simulink model "doa_no_gotos"  (R2013b)
settings: Solver=ode45  StartTime=0.0  StopTime=10.0  RelTol=1e-3
undefined symbols (not defined in the file or in its folder): calan_lib, comp_addsub
libraries: xbsIndex_r4 x1532, casper_library_misc x168, casper_library_delays x24
(part 1 of 16)
settings Model: Creator=root  LastModifiedBy=root

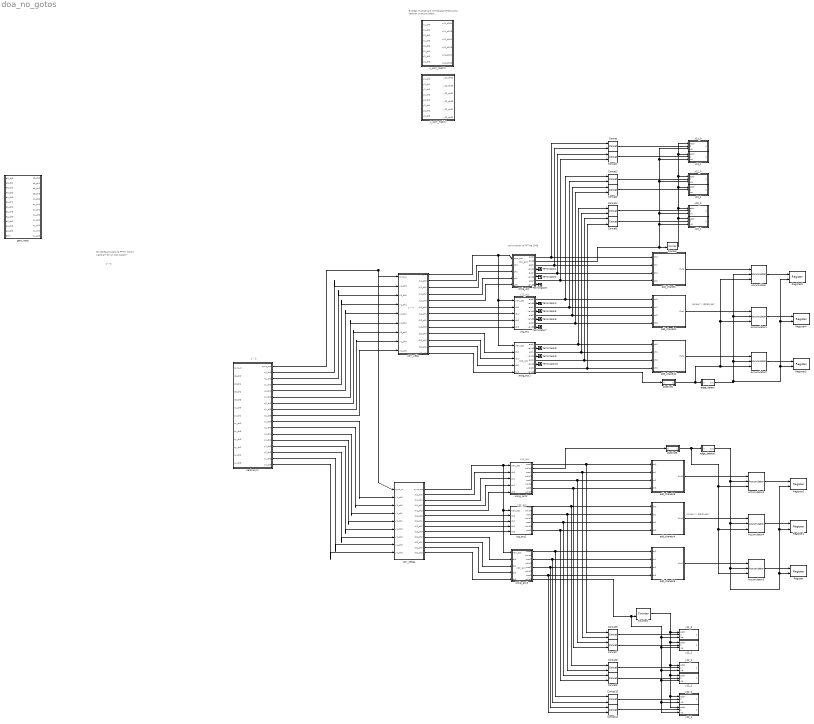
== system doa_no_gotos ==
  note: review!!! datatype!!
  note: x11_acc
  note: x12_acc
  note: x22_acc
  note: voy a tomar la FFT de 2048
  note: z^-7
  note: z^-2
  note: El diego multiplica e inmediatamente suma
      | todo en un acumulador..
  note: z^-3
  note: Es necesario para la FFT??
      | Como calibrar? en un solo canal??
  note: x11_acc
  note: x12_acc
  note: x22_acc
  note: review!!! datatype!!
  Accumulator{,1..5} (6 alike) : xbsIndex_r4/Accumulator  operation=Add  n_bits=64  overflow=Saturate  scale=1  rst=on  infoeditControl=reset for floating point data type must be asserted for a minimum of 2 cycles  hasbypass=off  en=on  latency=0  dbl_ovrd=off  msb_inp=100  msb=100  lsb=-100  use_behavioral_HDL=on  implementation=Fabric  block_type=accum
  Concat{,1..11} (12 alike) : xbsIndex_r4/Concat  num_inputs=2  dbl_ovrd=off  block_type=concat
  Counter : xbsIndex_r4/Counter  cnt_type=Free Running  cnt_to=Inf  operation=Up  start_count=0  cnt_by_val=1  arith_type=Unsigned  n_bits=9  bin_pt=0  load_pin=off  rst=on  en=on  explicit_period=on  period=1  dbl_ovrd=off  use_behavioral_HDL=off  implementation=Fabric  block_type=counter
  Counter1 : xbsIndex_r4/Counter  cnt_type=Free Running  cnt_to=Inf  operation=Up  start_count=0  cnt_by_val=1  arith_type=Unsigned  n_bits=9  bin_pt=0  load_pin=off  rst=on  en=on  explicit_period=on  period=1  dbl_ovrd=off  use_behavioral_HDL=off  implementation=Fabric  block_type=counter
  Register{,1..5} (6 alike) : xbsIndex_r4/Register  init=0  rst=off  en=on  dbl_ovrd=off  block_type=register
  Terminator{1..10} (10 alike) : Terminator
  add_chanels : Subsystem
  add_chanels1 : Subsystem
  add_chanels2 : Subsystem
  add_chanels3 : Subsystem
  add_chanels4 : Subsystem
  add_chanels5 : Subsystem
  centrosym : Subsystem
  corr_seba : Subsystem
  corr_seba1 : Subsystem
  edge_detect : Subsystem  AncestorBlock=casper_library_misc/edge_detect  mask(edge_detect){edge=Falling, polarity=Active High, x_in=[0 0.08 0.08 0.16 0.16 0.24 0.24 0.32 0.32 0.4], y_in=[-1 -1  1  1  1  1  1  1  1  1], x_out=[0.6 0.68 0.68 0.76 0.76 0.84 0.84 0.92 0.92 1], y_out=[-1 -1  1  1 -1 -1 -1 -1 -1 -1]}
      mask prompts: edge "Edge Type"; polarity "Output Polarity"; x_in "Input X Positions"; y_in "Input Y Positions"; x_out "Output X Positions"; y_out "Output Y Positions"
      mask help: Output is active for one-cycle after each edge of the specified type (i.e. rising, falling or both).
      mask init:
      | edge_detect_init(gcb,...
      |     'edge',edge,...
      |     'polarity',polarity,...
      |     'x_in',x_in,...
      |     'x_out',x_out,...
      |     'y_in',y_in,...
      |     'y_out',y_out);
      | 
      | x_in_num=str2num(getfield(getfield(get_param(gcb,'UserData'),'parameters'),'x_in'));
      | x_out_num=str2num(getfield(getfield(get_param(gcb,'UserData'),'parameters'),'x_out'));
      | y_in_num=str2num(getfield(getfield(get_param(gcb,'UserData'),'parameters'),'y_in'));
      | y_out_num=str2num(getfield(getfield(get_param(gcb,'UserData'),'parameters'),'y_out'));
      settings: AttributesFormatString=|
      | falling edges
      | active high
      mask Help: Output is active for one-cycle after each edge of the specified type (i.e. rising, falling, or both).  Latency is zero.
      mask TypeOptions edge: Rising | Falling | Both
      mask TypeOptions polarity: Active High | Active Low
      mask Display:
      | plot(x_in_num,0.5+y_in_num*0.2);
      | plot(x_out_num,0.5+y_out_num*0.2);
  edge_detect1 : Subsystem  AncestorBlock=casper_library_misc/edge_detect  mask(edge_detect){edge=Falling, polarity=Active High, x_in=[0 0.08 0.08 0.16 0.16 0.24 0.24 0.32 0.32 0.4], y_in=[-1 -1  1  1  1  1  1  1  1  1], x_out=[0.6 0.68 0.68 0.76 0.76 0.84 0.84 0.92 0.92 1], y_out=[-1 -1  1  1 -1 -1 -1 -1 -1 -1]}
      mask prompts: edge "Edge Type"; polarity "Output Polarity"; x_in "Input X Positions"; y_in "Input Y Positions"; x_out "Output X Positions"; y_out "Output Y Positions"
      mask help: Output is active for one-cycle after each edge of the specified type (i.e. rising, falling or both).
      mask init: same as doa_no_gotos/edge_detect
      settings: AttributesFormatString=|
      | falling edges
      | active high
      mask Help: Output is active for one-cycle after each edge of the specified type (i.e. rising, falling, or both).  Latency is zero.
      mask TypeOptions edge: Rising | Falling | Both
      mask TypeOptions polarity: Active High | Active Low
      mask Display:
      | plot(x_in_num,0.5+y_in_num*0.2);
      | plot(x_out_num,0.5+y_out_num*0.2);
  gain_input : Subsystem
  pipeline1 : Subsystem  AncestorBlock=casper_library_delays/pipeline  mask(pipeline){latency=9}
      mask help:
      | An explicitly laid-out delay line to avoid mapping to SRL16s
      | for use in pipelining to help achieve timing closure.
      mask init:
      | pipeline_init(gcb,'latency',latency);
      settings: AttributesFormatString=Latency = %<latency>
      mask Display:
      | port_label('input', 1, 'd');
      | port_label('output', 1, 'q');
      | disp(['Z^-', num2str(latency)]);
  pipeline5 : Subsystem  AncestorBlock=casper_library_delays/pipeline  mask(pipeline){latency=9}
      mask help:
      | An explicitly laid-out delay line to avoid mapping to SRL16s
      | for use in pipelining to help achieve timing closure.
      mask init:
      | pipeline_init(gcb,'latency',latency);
      settings: AttributesFormatString=Latency = %<latency>
      mask Display:
      | port_label('input', 1, 'd');
      | port_label('output', 1, 'q');
      | disp(['Z^-', num2str(latency)]);
  sig_acc : Subsystem
  sig_acc1 : Subsystem
  unsig_acc : Subsystem
  unsig_acc1 : Subsystem
  unsig_acc2 : Subsystem
  unsig_acc3 : Subsystem
  x11_0 : Subsystem  Tag=xps:bram  AncestorBlock=xps_library/Shared_BRAM  mask{arith_type=Unsigned, addr_width=9, data_width=64, reg_prim_output=off, reg_core_output=off, optimization=Minimum_Area, data_bin_pt=0, init_vals=[0:2^10-1], sample_rate=1}
      mask prompts: arith_type "Output Data Type"; addr_width "Address width"; data_width "Data Width"; reg_prim_output "Register Primitive Output"; reg_core_output "Register Core Output"; data_bin_pt "Data Binary Point"; init_vals "Initial values (simulation only)"; sample_rate "Sample rate"
      mask init:
      | shared_bram_mask;
      mask TypeOptions arith_type: Unsigned | Signed  (2's comp)
      mask TypeOptions data_width: 8 | 16 | 32 | 64 | 128
      mask TypeOptions optimization: Minimum_Area | Low_Power
  x11_1 : Subsystem  Tag=xps:bram  AncestorBlock=xps_library/Shared_BRAM  mask{arith_type=Unsigned, addr_width=9, data_width=64, reg_prim_output=off, reg_core_output=off, optimization=Minimum_Area, data_bin_pt=0, init_vals=[0:2^10-1], sample_rate=1}
      mask prompts: arith_type "Output Data Type"; addr_width "Address width"; data_width "Data Width"; reg_prim_output "Register Primitive Output"; reg_core_output "Register Core Output"; data_bin_pt "Data Binary Point"; init_vals "Initial values (simulation only)"; sample_rate "Sample rate"
      mask init:
      | shared_bram_mask;
      mask TypeOptions arith_type: Unsigned | Signed  (2's comp)
      mask TypeOptions data_width: 8 | 16 | 32 | 64 | 128
      mask TypeOptions optimization: Minimum_Area | Low_Power
  x12_0 : Subsystem  Tag=xps:bram  AncestorBlock=xps_library/Shared_BRAM  mask{arith_type=Unsigned, addr_width=9, data_width=64, reg_prim_output=off, reg_core_output=off, optimization=Minimum_Area, data_bin_pt=0, init_vals=[0:2^10-1], sample_rate=1}
      mask prompts: arith_type "Output Data Type"; addr_width "Address width"; data_width "Data Width"; reg_prim_output "Register Primitive Output"; reg_core_output "Register Core Output"; data_bin_pt "Data Binary Point"; init_vals "Initial values (simulation only)"; sample_rate "Sample rate"
      mask init:
      | shared_bram_mask;
      mask TypeOptions arith_type: Unsigned | Signed  (2's comp)
      mask TypeOptions data_width: 8 | 16 | 32 | 64 | 128
      mask TypeOptions optimization: Minimum_Area | Low_Power
  x12_1 : Subsystem  Tag=xps:bram  AncestorBlock=xps_library/Shared_BRAM  mask{arith_type=Unsigned, addr_width=9, data_width=64, reg_prim_output=off, reg_core_output=off, optimization=Minimum_Area, data_bin_pt=0, init_vals=[0:2^10-1], sample_rate=1}
      mask prompts: arith_type "Output Data Type"; addr_width "Address width"; data_width "Data Width"; reg_prim_output "Register Primitive Output"; reg_core_output "Register Core Output"; data_bin_pt "Data Binary Point"; init_vals "Initial values (simulation only)"; sample_rate "Sample rate"
      mask init:
      | shared_bram_mask;
      mask TypeOptions arith_type: Unsigned | Signed  (2's comp)
      mask TypeOptions data_width: 8 | 16 | 32 | 64 | 128
      mask TypeOptions optimization: Minimum_Area | Low_Power
  x22_0 : Subsystem  Tag=xps:bram  AncestorBlock=xps_library/Shared_BRAM  mask{arith_type=Unsigned, addr_width=9, data_width=64, reg_prim_output=off, reg_core_output=off, optimization=Minimum_Area, data_bin_pt=0, init_vals=[0:2^10-1], sample_rate=1}
      mask prompts: arith_type "Output Data Type"; addr_width "Address width"; data_width "Data Width"; reg_prim_output "Register Primitive Output"; reg_core_output "Register Core Output"; data_bin_pt "Data Binary Point"; init_vals "Initial values (simulation only)"; sample_rate "Sample rate"
      mask init:
      | shared_bram_mask;
      mask TypeOptions arith_type: Unsigned | Signed  (2's comp)
      mask TypeOptions data_width: 8 | 16 | 32 | 64 | 128
      mask TypeOptions optimization: Minimum_Area | Low_Power
  x22_1 : Subsystem  Tag=xps:bram  AncestorBlock=xps_library/Shared_BRAM  mask{arith_type=Unsigned, addr_width=9, data_width=64, reg_prim_output=off, reg_core_output=off, optimization=Minimum_Area, data_bin_pt=0, init_vals=[0:2^10-1], sample_rate=1}
      mask prompts: arith_type "Output Data Type"; addr_width "Address width"; data_width "Data Width"; reg_prim_output "Register Primitive Output"; reg_core_output "Register Core Output"; data_bin_pt "Data Binary Point"; init_vals "Initial values (simulation only)"; sample_rate "Sample rate"
      mask init:
      | shared_bram_mask;
      mask TypeOptions arith_type: Unsigned | Signed  (2's comp)
      mask TypeOptions data_width: 8 | 16 | 32 | 64 | 128
      mask TypeOptions optimization: Minimum_Area | Low_Power
  x_corr_matrix : Subsystem
  y11_0 : Subsystem  Tag=xps:bram  AncestorBlock=xps_library/Shared_BRAM  mask{arith_type=Unsigned, addr_width=9, data_width=64, reg_prim_output=off, reg_core_output=off, optimization=Minimum_Area, data_bin_pt=0, init_vals=[0:2^10-1], sample_rate=1}
      mask prompts: arith_type "Output Data Type"; addr_width "Address width"; data_width "Data Width"; reg_prim_output "Register Primitive Output"; reg_core_output "Register Core Output"; data_bin_pt "Data Binary Point"; init_vals "Initial values (simulation only)"; sample_rate "Sample rate"
      mask init:
      | shared_bram_mask;
      mask TypeOptions arith_type: Unsigned | Signed  (2's comp)
      mask TypeOptions data_width: 8 | 16 | 32 | 64 | 128
      mask TypeOptions optimization: Minimum_Area | Low_Power
  y11_1 : Subsystem  Tag=xps:bram  AncestorBlock=xps_library/Shared_BRAM  mask{arith_type=Unsigned, addr_width=9, data_width=64, reg_prim_output=off, reg_core_output=off, optimization=Minimum_Area, data_bin_pt=0, init_vals=[0:2^10-1], sample_rate=1}
      mask prompts: arith_type "Output Data Type"; addr_width "Address width"; data_width "Data Width"; reg_prim_output "Register Primitive Output"; reg_core_output "Register Core Output"; data_bin_pt "Data Binary Point"; init_vals "Initial values (simulation only)"; sample_rate "Sample rate"
      mask init:
      | shared_bram_mask;
      mask TypeOptions arith_type: Unsigned | Signed  (2's comp)
      mask TypeOptions data_width: 8 | 16 | 32 | 64 | 128
      mask TypeOptions optimization: Minimum_Area | Low_Power
  y12_0 : Subsystem  Tag=xps:bram  AncestorBlock=xps_library/Shared_BRAM  mask{arith_type=Unsigned, addr_width=9, data_width=64, reg_prim_output=off, reg_core_output=off, optimization=Minimum_Area, data_bin_pt=0, init_vals=[0:2^10-1], sample_rate=1}
      mask prompts: arith_type "Output Data Type"; addr_width "Address width"; data_width "Data Width"; reg_prim_output "Register Primitive Output"; reg_core_output "Register Core Output"; data_bin_pt "Data Binary Point"; init_vals "Initial values (simulation only)"; sample_rate "Sample rate"
      mask init:
      | shared_bram_mask;
      mask TypeOptions arith_type: Unsigned | Signed  (2's comp)
      mask TypeOptions data_width: 8 | 16 | 32 | 64 | 128
      mask TypeOptions optimization: Minimum_Area | Low_Power
  y12_1 : Subsystem  Tag=xps:bram  AncestorBlock=xps_library/Shared_BRAM  mask{arith_type=Unsigned, addr_width=9, data_width=64, reg_prim_output=off, reg_core_output=off, optimization=Minimum_Area, data_bin_pt=0, init_vals=[0:2^10-1], sample_rate=1}
      mask prompts: arith_type "Output Data Type"; addr_width "Address width"; data_width "Data Width"; reg_prim_output "Register Primitive Output"; reg_core_output "Register Core Output"; data_bin_pt "Data Binary Point"; init_vals "Initial values (simulation only)"; sample_rate "Sample rate"
      mask init:
      | shared_bram_mask;
      mask TypeOptions arith_type: Unsigned | Signed  (2's comp)
      mask TypeOptions data_width: 8 | 16 | 32 | 64 | 128
      mask TypeOptions optimization: Minimum_Area | Low_Power
  y22_0 : Subsystem  Tag=xps:bram  AncestorBlock=xps_library/Shared_BRAM  mask{arith_type=Unsigned, addr_width=9, data_width=64, reg_prim_output=off, reg_core_output=off, optimization=Minimum_Area, data_bin_pt=0, init_vals=[0:2^10-1], sample_rate=1}
      mask prompts: arith_type "Output Data Type"; addr_width "Address width"; data_width "Data Width"; reg_prim_output "Register Primitive Output"; reg_core_output "Register Core Output"; data_bin_pt "Data Binary Point"; init_vals "Initial values (simulation only)"; sample_rate "Sample rate"
      mask init:
      | shared_bram_mask;
      mask TypeOptions arith_type: Unsigned | Signed  (2's comp)
      mask TypeOptions data_width: 8 | 16 | 32 | 64 | 128
      mask TypeOptions optimization: Minimum_Area | Low_Power
  y22_1 : Subsystem  Tag=xps:bram  AncestorBlock=xps_library/Shared_BRAM  mask{arith_type=Unsigned, addr_width=9, data_width=64, reg_prim_output=off, reg_core_output=off, optimization=Minimum_Area, data_bin_pt=0, init_vals=[0:2^10-1], sample_rate=1}
      mask prompts: arith_type "Output Data Type"; addr_width "Address width"; data_width "Data Width"; reg_prim_output "Register Primitive Output"; reg_core_output "Register Core Output"; data_bin_pt "Data Binary Point"; init_vals "Initial values (simulation only)"; sample_rate "Sample rate"
      mask init:
      | shared_bram_mask;
      mask TypeOptions arith_type: Unsigned | Signed  (2's comp)
      mask TypeOptions data_width: 8 | 16 | 32 | 64 | 128
      mask TypeOptions optimization: Minimum_Area | Low_Power
  y_corr_matrix : Subsystem
  wires:
  corr_seba/5(r11_ch3) -> unsig_acc/5(ch3)
  corr_seba/2(r11_ch0) -> unsig_acc/2(ch0)
  corr_seba/4(r11_ch2) -> unsig_acc/4(ch2)
  corr_seba/3(r11_ch1) -> unsig_acc/3(ch1)
  corr_seba/1(sync_out) -> unsig_acc/1(new_acc), unsig_acc1/1(new_acc), sig_acc/1(new_acc)
  corr_seba/6(r12_ch0) -> sig_acc/2(ch0)
  corr_seba/7(r12_ch1) -> sig_acc/3(ch1)
  corr_seba/8(r12_ch2) -> sig_acc/4(ch2)
  corr_seba/9(r12_ch3) -> sig_acc/5(ch3)
  corr_seba/10(r22_ch0) -> unsig_acc1/2(ch0)
  corr_seba/13(r22_ch3) -> unsig_acc1/5(ch3)
  corr_seba/12(r22_ch2) -> unsig_acc1/4(ch2)
  corr_seba/11(r22_ch1) -> unsig_acc1/3(ch1)
  centrosym/1(sync_out) -> corr_seba1/1(sync_in), corr_seba/1(sync_in)
  centrosym/2(x1_ch0) -> corr_seba/2(x1_ch0)
  centrosym/3(x2_ch0) -> corr_seba/3(x2_ch0)
  centrosym/4(x1_ch1) -> corr_seba/4(x1_ch1)
  centrosym/5(x2_ch1) -> corr_seba/5(x2_ch1)
  centrosym/6(x1_ch2) -> corr_seba/6(x1_ch2)
  centrosym/7(x2_ch2) -> corr_seba/7(x2_ch2)
  centrosym/8(x1_ch3) -> corr_seba/8(x1_ch3)
  centrosym/9(x2_ch3) -> corr_seba/9(x2_ch3)
  corr_seba1/5(r11_ch3) -> unsig_acc2/5(ch3)
  corr_seba1/2(r11_ch0) -> unsig_acc2/2(ch0)
  corr_seba1/4(r11_ch2) -> unsig_acc2/4(ch2)
  corr_seba1/3(r11_ch1) -> unsig_acc2/3(ch1)
  corr_seba1/1(sync_out) -> unsig_acc3/1(new_acc), sig_acc1/1(new_acc), unsig_acc2/1(new_acc)
  corr_seba1/6(r12_ch0) -> sig_acc1/2(ch0)
  corr_seba1/7(r12_ch1) -> sig_acc1/3(ch1)
  corr_seba1/8(r12_ch2) -> sig_acc1/4(ch2)
  corr_seba1/9(r12_ch3) -> sig_acc1/5(ch3)
  corr_seba1/10(r22_ch0) -> unsig_acc3/2(ch0)
  corr_seba1/13(r22_ch3) -> unsig_acc3/5(ch3)
  corr_seba1/12(r22_ch2) -> unsig_acc3/4(ch2)
  corr_seba1/11(r22_ch1) -> unsig_acc3/3(ch1)
  centrosym/10(y1_ch0) -> corr_seba1/2(y1_ch0)
  centrosym/11(y2_ch0) -> corr_seba1/3(y2_ch0)
  centrosym/12(y1_ch1) -> corr_seba1/4(y1_ch1)
  centrosym/13(y2_ch1) -> corr_seba1/5(y2_ch1)
  centrosym/14(y1_ch2) -> corr_seba1/6(y1_ch2)
  centrosym/15(y2_ch2) -> corr_seba1/7(y2_ch2)
  centrosym/16(y1_ch3) -> corr_seba1/8(y1_ch3)
  centrosym/17(y2_ch3) -> corr_seba1/9(y2_ch3)
  pipeline1/1(q) -> edge_detect/1(in), Accumulator2/3, Accumulator1/3, Accumulator/3
  edge_detect/1(out) -> Register5/2, Register4/2, Register3/2, Accumulator2/2, Accumulator1/2, Accumulator/2
  unsig_acc1/8(valid3) -> pipeline1/1(d)
  unsig_acc/1(acc0) -> Concat/1, add_chanels/1(ch0)
  unsig_acc/3(acc1) -> Concat/2, add_chanels/2(ch1)
  unsig_acc/5(acc2) -> Concat1/1, add_chanels/3(ch2)
  unsig_acc/7(acc3) -> Concat1/2, add_chanels/4(ch3)
  add_chanels/1(Out1) -> Accumulator/1
  sig_acc/1(acc0) -> Concat2/1, add_chanels1/1(ch0)
  sig_acc/3(acc1) -> Concat2/2, add_chanels1/2(ch1)
  sig_acc/5(acc2) -> Concat3/1, add_chanels1/3(ch2)
  sig_acc/7(acc3) -> Concat3/2, add_chanels1/4(ch3)
  unsig_acc1/1(acc0) -> Concat4/1, add_chanels2/1(ch0)
  unsig_acc1/3(acc1) -> Concat4/2, add_chanels2/2(ch1)
  unsig_acc1/5(acc2) -> Concat5/1, add_chanels2/3(ch2)
  unsig_acc1/7(acc3) -> add_chanels2/4(ch3), Concat5/2
  add_chanels1/1(Out1) -> Accumulator1/1
  add_chanels2/1(Out1) -> Accumulator2/1
  unsig_acc/2(valid0) -> x22_0/3(we), x11_1/3(we), x11_0/3(we), x12_0/3(we), x22_1/3(we), Counter/2
  unsig_acc/4(valid1) -> Terminator1/1
  unsig_acc/6(valid2) -> Terminator2/1
  unsig_acc/8(valid3) -> Terminator3/1
  sig_acc/2(valid0) -> Terminator4/1
  sig_acc/4(valid1) -> Terminator5/1
  sig_acc/6(valid2) -> Terminator6/1
  sig_acc/8(valid3) -> Terminator7/1
  unsig_acc1/2(valid0) -> Terminator8/1
  unsig_acc1/4(valid1) -> Terminator9/1
  unsig_acc1/6(valid2) -> Terminator10/1
  pipeline5/1(q) -> Accumulator5/3, Accumulator4/3, Accumulator3/3, edge_detect1/1(in)
  edge_detect1/1(out) -> Register/2, Register1/2, Register2/2, Accumulator5/2, Accumulator4/2, Accumulator3/2
  unsig_acc2/2(valid0) -> pipeline5/1(d)
  unsig_acc2/1(acc0) -> Concat6/1, add_chanels3/1(ch0)
  unsig_acc2/3(acc1) -> Concat6/2, add_chanels3/2(ch1)
  unsig_acc2/5(acc2) -> Concat7/1, add_chanels3/3(ch2)
  unsig_acc2/7(acc3) -> Concat7/2, add_chanels3/4(ch3)
  add_chanels3/1(Out1) -> Accumulator3/1
  sig_acc1/1(acc0) -> Concat8/1, add_chanels4/1(ch0)
  sig_acc1/3(acc1) -> Concat8/2, add_chanels4/2(ch1)
  sig_acc1/5(acc2) -> Concat9/1, add_chanels4/3(ch2)
  sig_acc1/7(acc3) -> Concat9/2, add_chanels4/4(ch3)
  unsig_acc3/1(acc0) -> Concat10/1, add_chanels5/1(ch0)
  unsig_acc3/3(acc1) -> Concat10/2, add_chanels5/2(ch1)
  unsig_acc3/5(acc2) -> Concat11/1, add_chanels5/3(ch2)
  unsig_acc3/7(acc3) -> add_chanels5/4(ch3), Concat11/2
  add_chanels4/1(Out1) -> Accumulator4/1
  add_chanels5/1(Out1) -> Accumulator5/1
  Accumulator5/1 -> Register/1
  Accumulator4/1 -> Register1/1
  Accumulator3/1 -> Register2/1
  Accumulator2/1 -> Register3/1
  Accumulator1/1 -> Register4/1
  Accumulator/1 -> Register5/1
  Concat1/1 -> x11_1/2(data_in)
  Concat/1 -> x11_0/2(data_in)
  Concat2/1 -> x12_0/2(data_in)
  Concat3/1 -> x12_1/2(data_in)
  Concat4/1 -> x22_0/2(data_in)
  Concat5/1 -> x22_1/2(data_in)
  Counter/1 -> x12_1/1(addr), x11_0/1(addr), x11_1/1(addr), x12_0/1(addr), x22_0/1(addr), x22_1/1(addr)
  Concat7/1 -> y11_1/2(data_in)
  Concat6/1 -> y11_0/2(data_in)
  Concat8/1 -> y12_0/2(data_in)
  Concat9/1 -> y12_1/2(data_in)
  Concat10/1 -> y22_0/2(data_in)
  Concat11/1 -> y22_1/2(data_in)
  unsig_acc3/8(valid3) -> y12_1/3(we), y22_1/3(we), y22_0/3(we), y12_0/3(we), y11_1/3(we), y11_0/3(we), Counter1/2
  Counter1/1 -> y11_1/1(addr), y12_1/1(addr), y22_0/1(addr), y22_1/1(addr), y12_0/1(addr), y11_0/1(addr)

== system doa_no_gotos/add_chanels ==
  ch0 : Inport
  ch1 : Inport  Port=2
  ch2 : Inport  Port=3
  ch3 : Inport  Port=4
  AddSub : xbsIndex_r4/AddSub  mode=Addition  use_carryin=off  use_carryout=off  en=off  latency=2  precision=User Defined  arith_type=Unsigned  n_bits=64  bin_pt=35  quantization=Truncate  overflow=Wrap  dbl_ovrd=off  use_behavioral_HDL=off  hw_selection=Fabric  pipelined=off  block_type=addsub
  AddSub1 : xbsIndex_r4/AddSub  mode=Addition  use_carryin=off  use_carryout=off  en=off  latency=2  precision=User Defined  arith_type=Unsigned  n_bits=64  bin_pt=35  quantization=Truncate  overflow=Wrap  dbl_ovrd=off  use_behavioral_HDL=off  hw_selection=Fabric  pipelined=off  block_type=addsub
  AddSub2 : xbsIndex_r4/AddSub  mode=Addition  use_carryin=off  use_carryout=off  en=off  latency=2  precision=User Defined  arith_type=Unsigned  n_bits=64  bin_pt=35  quantization=Truncate  overflow=Wrap  dbl_ovrd=off  use_behavioral_HDL=off  hw_selection=Fabric  pipelined=off  block_type=addsub
  pipeline243 : Subsystem  AncestorBlock=casper_library_delays/pipeline  mask(pipeline){latency=2}
      mask help:
      | An explicitly laid-out delay line to avoid mapping to SRL16s
      | for use in pipelining to help achieve timing closure.
      mask init:
      | pipeline_init(gcb,'latency',latency);
      settings: AttributesFormatString=Latency = %<latency>
      mask Display:
      | port_label('input', 1, 'd');
      | port_label('output', 1, 'q');
      | disp(['Z^-', num2str(latency)]);
  pipeline244 : Subsystem  AncestorBlock=casper_library_delays/pipeline  mask(pipeline){latency=2}
      mask help:
      | An explicitly laid-out delay line to avoid mapping to SRL16s
      | for use in pipelining to help achieve timing closure.
      mask init:
      | pipeline_init(gcb,'latency',latency);
      settings: AttributesFormatString=Latency = %<latency>
      mask Display:
      | port_label('input', 1, 'd');
      | port_label('output', 1, 'q');
      | disp(['Z^-', num2str(latency)]);
  pipeline{87,245,247,249} (4 alike) : casper_library_delays/pipeline  latency=3
      settings: AttributesFormatString=Latency = %<latency>
  pipeline246 : Subsystem  AncestorBlock=casper_library_delays/pipeline  mask(pipeline){latency=2}
      mask help:
      | An explicitly laid-out delay line to avoid mapping to SRL16s
      | for use in pipelining to help achieve timing closure.
      mask init:
      | pipeline_init(gcb,'latency',latency);
      settings: AttributesFormatString=Latency = %<latency>
      mask Display:
      | port_label('input', 1, 'd');
      | port_label('output', 1, 'q');
      | disp(['Z^-', num2str(latency)]);
  pipeline248 : Subsystem  AncestorBlock=casper_library_delays/pipeline  mask(pipeline){latency=2}
      mask help:
      | An explicitly laid-out delay line to avoid mapping to SRL16s
      | for use in pipelining to help achieve timing closure.
      mask init:
      | pipeline_init(gcb,'latency',latency);
      settings: AttributesFormatString=Latency = %<latency>
      mask Display:
      | port_label('input', 1, 'd');
      | port_label('output', 1, 'q');
      | disp(['Z^-', num2str(latency)]);
  Out1 : Outport
  wires:
  pipeline244/1(q) -> pipeline245/1
  pipeline243/1(q) -> pipeline87/1
  ch0/1 -> pipeline248/1(d)
  pipeline247/1 -> AddSub/2
  ch2/1 -> pipeline244/1(d)
  pipeline249/1 -> AddSub/1
  AddSub/1 -> AddSub2/1
  pipeline246/1(q) -> pipeline247/1
  pipeline248/1(q) -> pipeline249/1
  pipeline245/1 -> AddSub1/1
  AddSub2/1 -> Out1/1
  pipeline87/1 -> AddSub1/2
  AddSub1/1 -> AddSub2/2
  ch1/1 -> pipeline246/1(d)
  ch3/1 -> pipeline243/1(d)

== system doa_no_gotos/add_chanels1 ==
  ch0 : Inport
  ch1 : Inport  Port=2
  ch2 : Inport  Port=3
  ch3 : Inport  Port=4
  AddSub : xbsIndex_r4/AddSub  mode=Addition  use_carryin=off  use_carryout=off  en=off  latency=2  precision=User Defined  arith_type=Unsigned  n_bits=64  bin_pt=35  quantization=Truncate  overflow=Wrap  dbl_ovrd=off  use_behavioral_HDL=off  hw_selection=Fabric  pipelined=off  block_type=addsub
  AddSub1 : xbsIndex_r4/AddSub  mode=Addition  use_carryin=off  use_carryout=off  en=off  latency=2  precision=User Defined  arith_type=Unsigned  n_bits=64  bin_pt=35  quantization=Truncate  overflow=Wrap  dbl_ovrd=off  use_behavioral_HDL=off  hw_selection=Fabric  pipelined=off  block_type=addsub
  AddSub2 : xbsIndex_r4/AddSub  mode=Addition  use_carryin=off  use_carryout=off  en=off  latency=2  precision=User Defined  arith_type=Unsigned  n_bits=64  bin_pt=35  quantization=Truncate  overflow=Wrap  dbl_ovrd=off  use_behavioral_HDL=off  hw_selection=Fabric  pipelined=off  block_type=addsub
  pipeline243 : Subsystem  AncestorBlock=casper_library_delays/pipeline  mask(pipeline){latency=2}
      mask help:
      | An explicitly laid-out delay line to avoid mapping to SRL16s
      | for use in pipelining to help achieve timing closure.
      mask init:
      | pipeline_init(gcb,'latency',latency);
      settings: AttributesFormatString=Latency = %<latency>
      mask Display:
      | port_label('input', 1, 'd');
      | port_label('output', 1, 'q');
      | disp(['Z^-', num2str(latency)]);
  pipeline244 : Subsystem  AncestorBlock=casper_library_delays/pipeline  mask(pipeline){latency=2}
      mask help:
      | An explicitly laid-out delay line to avoid mapping to SRL16s
      | for use in pipelining to help achieve timing closure.
      mask init:
      | pipeline_init(gcb,'latency',latency);
      settings: AttributesFormatString=Latency = %<latency>
      mask Display:
      | port_label('input', 1, 'd');
      | port_label('output', 1, 'q');
      | disp(['Z^-', num2str(latency)]);
  pipeline{87,245,247,249} (4 alike) : casper_library_delays/pipeline  latency=3
      settings: AttributesFormatString=Latency = %<latency>
  pipeline246 : Subsystem  AncestorBlock=casper_library_delays/pipeline  mask(pipeline){latency=2}
      mask help:
      | An explicitly laid-out delay line to avoid mapping to SRL16s
      | for use in pipelining to help achieve timing closure.
      mask init:
      | pipeline_init(gcb,'latency',latency);
      settings: AttributesFormatString=Latency = %<latency>
      mask Display:
      | port_label('input', 1, 'd');
      | port_label('output', 1, 'q');
      | disp(['Z^-', num2str(latency)]);
  pipeline248 : Subsystem  AncestorBlock=casper_library_delays/pipeline  mask(pipeline){latency=2}
      mask help:
      | An explicitly laid-out delay line to avoid mapping to SRL16s
      | for use in pipelining to help achieve timing closure.
      mask init:
      | pipeline_init(gcb,'latency',latency);
      settings: AttributesFormatString=Latency = %<latency>
      mask Display:
      | port_label('input', 1, 'd');
      | port_label('output', 1, 'q');
      | disp(['Z^-', num2str(latency)]);
  Out1 : Outport
  wires:
  pipeline244/1(q) -> pipeline245/1
  pipeline243/1(q) -> pipeline87/1
  ch0/1 -> pipeline248/1(d)
  pipeline247/1 -> AddSub/2
  ch2/1 -> pipeline244/1(d)
  pipeline249/1 -> AddSub/1
  AddSub/1 -> AddSub2/1
  pipeline246/1(q) -> pipeline247/1
  pipeline248/1(q) -> pipeline249/1
  pipeline245/1 -> AddSub1/1
  AddSub2/1 -> Out1/1
  pipeline87/1 -> AddSub1/2
  AddSub1/1 -> AddSub2/2
  ch1/1 -> pipeline246/1(d)
  ch3/1 -> pipeline243/1(d)

== system doa_no_gotos/add_chanels2 ==
  ch0 : Inport
  ch1 : Inport  Port=2
  ch2 : Inport  Port=3
  ch3 : Inport  Port=4
  AddSub : xbsIndex_r4/AddSub  mode=Addition  use_carryin=off  use_carryout=off  en=off  latency=2  precision=User Defined  arith_type=Unsigned  n_bits=64  bin_pt=35  quantization=Truncate  overflow=Wrap  dbl_ovrd=off  use_behavioral_HDL=off  hw_selection=Fabric  pipelined=off  block_type=addsub
  AddSub1 : xbsIndex_r4/AddSub  mode=Addition  use_carryin=off  use_carryout=off  en=off  latency=2  precision=User Defined  arith_type=Unsigned  n_bits=64  bin_pt=35  quantization=Truncate  overflow=Wrap  dbl_ovrd=off  use_behavioral_HDL=off  hw_selection=Fabric  pipelined=off  block_type=addsub
  AddSub2 : xbsIndex_r4/AddSub  mode=Addition  use_carryin=off  use_carryout=off  en=off  latency=2  precision=User Defined  arith_type=Unsigned  n_bits=64  bin_pt=35  quantization=Truncate  overflow=Wrap  dbl_ovrd=off  use_behavioral_HDL=off  hw_selection=Fabric  pipelined=off  block_type=addsub
  pipeline243 : Subsystem  AncestorBlock=casper_library_delays/pipeline  mask(pipeline){latency=2}
      mask help:
      | An explicitly laid-out delay line to avoid mapping to SRL16s
      | for use in pipelining to help achieve timing closure.
      mask init:
      | pipeline_init(gcb,'latency',latency);
      settings: AttributesFormatString=Latency = %<latency>
      mask Display:
      | port_label('input', 1, 'd');
      | port_label('output', 1, 'q');
      | disp(['Z^-', num2str(latency)]);
  pipeline244 : Subsystem  AncestorBlock=casper_library_delays/pipeline  mask(pipeline){latency=2}
      mask help:
      | An explicitly laid-out delay line to avoid mapping to SRL16s
      | for use in pipelining to help achieve timing closure.
      mask init:
      | pipeline_init(gcb,'latency',latency);
      settings: AttributesFormatString=Latency = %<latency>
      mask Display:
      | port_label('input', 1, 'd');
      | port_label('output', 1, 'q');
      | disp(['Z^-', num2str(latency)]);
  pipeline{87,245,247,249} (4 alike) : casper_library_delays/pipeline  latency=3
      settings: AttributesFormatString=Latency = %<latency>
  pipeline246 : Subsystem  AncestorBlock=casper_library_delays/pipeline  mask(pipeline){latency=2}
      mask help:
      | An explicitly laid-out delay line to avoid mapping to SRL16s
      | for use in pipelining to help achieve timing closure.
      mask init:
      | pipeline_init(gcb,'latency',latency);
      settings: AttributesFormatString=Latency = %<latency>
      mask Display:
      | port_label('input', 1, 'd');
      | port_label('output', 1, 'q');
      | disp(['Z^-', num2str(latency)]);
  pipeline248 : Subsystem  AncestorBlock=casper_library_delays/pipeline  mask(pipeline){latency=2}
      mask help:
      | An explicitly laid-out delay line to avoid mapping to SRL16s
      | for use in pipelining to help achieve timing closure.
      mask init:
      | pipeline_init(gcb,'latency',latency);
      settings: AttributesFormatString=Latency = %<latency>
      mask Display:
      | port_label('input', 1, 'd');
      | port_label('output', 1, 'q');
      | disp(['Z^-', num2str(latency)]);
  Out1 : Outport
  wires:
  pipeline244/1(q) -> pipeline245/1
  pipeline243/1(q) -> pipeline87/1
  ch0/1 -> pipeline248/1(d)
  pipeline247/1 -> AddSub/2
  ch2/1 -> pipeline244/1(d)
  pipeline249/1 -> AddSub/1
  AddSub/1 -> AddSub2/1
  pipeline246/1(q) -> pipeline247/1
  pipeline248/1(q) -> pipeline249/1
  pipeline245/1 -> AddSub1/1
  AddSub2/1 -> Out1/1
  pipeline87/1 -> AddSub1/2
  AddSub1/1 -> AddSub2/2
  ch1/1 -> pipeline246/1(d)
  ch3/1 -> pipeline243/1(d)

== system doa_no_gotos/add_chanels3 ==
  ch0 : Inport
  ch1 : Inport  Port=2
  ch2 : Inport  Port=3
  ch3 : Inport  Port=4
  AddSub : xbsIndex_r4/AddSub  mode=Addition  use_carryin=off  use_carryout=off  en=off  latency=2  precision=User Defined  arith_type=Unsigned  n_bits=64  bin_pt=35  quantization=Truncate  overflow=Wrap  dbl_ovrd=off  use_behavioral_HDL=off  hw_selection=Fabric  pipelined=off  block_type=addsub
  AddSub1 : xbsIndex_r4/AddSub  mode=Addition  use_carryin=off  use_carryout=off  en=off  latency=2  precision=User Defined  arith_type=Unsigned  n_bits=64  bin_pt=35  quantization=Truncate  overflow=Wrap  dbl_ovrd=off  use_behavioral_HDL=off  hw_selection=Fabric  pipelined=off  block_type=addsub
  AddSub2 : xbsIndex_r4/AddSub  mode=Addition  use_carryin=off  use_carryout=off  en=off  latency=2  precision=User Defined  arith_type=Unsigned  n_bits=64  bin_pt=35  quantization=Truncate  overflow=Wrap  dbl_ovrd=off  use_behavioral_HDL=off  hw_selection=Fabric  pipelined=off  block_type=addsub
  pipeline243 : Subsystem  AncestorBlock=casper_library_delays/pipeline  mask(pipeline){latency=2}
      mask help:
      | An explicitly laid-out delay line to avoid mapping to SRL16s
      | for use in pipelining to help achieve timing closure.
      mask init:
      | pipeline_init(gcb,'latency',latency);
      settings: AttributesFormatString=Latency = %<latency>
      mask Display:
      | port_label('input', 1, 'd');
      | port_label('output', 1, 'q');
      | disp(['Z^-', num2str(latency)]);
  pipeline244 : Subsystem  AncestorBlock=casper_library_delays/pipeline  mask(pipeline){latency=2}
      mask help:
      | An explicitly laid-out delay line to avoid mapping to SRL16s
      | for use in pipelining to help achieve timing closure.
      mask init:
      | pipeline_init(gcb,'latency',latency);
      settings: AttributesFormatString=Latency = %<latency>
      mask Display:
      | port_label('input', 1, 'd');
      | port_label('output', 1, 'q');
      | disp(['Z^-', num2str(latency)]);
  pipeline{87,245,247,249} (4 alike) : casper_library_delays/pipeline  latency=3
      settings: AttributesFormatString=Latency = %<latency>
  pipeline246 : Subsystem  AncestorBlock=casper_library_delays/pipeline  mask(pipeline){latency=2}
      mask help:
      | An explicitly laid-out delay line to avoid mapping to SRL16s
      | for use in pipelining to help achieve timing closure.
      mask init:
      | pipeline_init(gcb,'latency',latency);
      settings: AttributesFormatString=Latency = %<latency>
      mask Display:
      | port_label('input', 1, 'd');
      | port_label('output', 1, 'q');
      | disp(['Z^-', num2str(latency)]);
  pipeline248 : Subsystem  AncestorBlock=casper_library_delays/pipeline  mask(pipeline){latency=2}
      mask help:
      | An explicitly laid-out delay line to avoid mapping to SRL16s
      | for use in pipelining to help achieve timing closure.
      mask init:
      | pipeline_init(gcb,'latency',latency);
      settings: AttributesFormatString=Latency = %<latency>
      mask Display:
      | port_label('input', 1, 'd');
      | port_label('output', 1, 'q');
      | disp(['Z^-', num2str(latency)]);
  Out1 : Outport
  wires:
  pipeline244/1(q) -> pipeline245/1
  pipeline243/1(q) -> pipeline87/1
  ch0/1 -> pipeline248/1(d)
  pipeline247/1 -> AddSub/2
  ch2/1 -> pipeline244/1(d)
  pipeline249/1 -> AddSub/1
  AddSub/1 -> AddSub2/1
  pipeline246/1(q) -> pipeline247/1
  pipeline248/1(q) -> pipeline249/1
  pipeline245/1 -> AddSub1/1
  AddSub2/1 -> Out1/1
  pipeline87/1 -> AddSub1/2
  AddSub1/1 -> AddSub2/2
  ch1/1 -> pipeline246/1(d)
  ch3/1 -> pipeline243/1(d)

== system doa_no_gotos/add_chanels4 ==
  ch0 : Inport
  ch1 : Inport  Port=2
  ch2 : Inport  Port=3
  ch3 : Inport  Port=4
  AddSub : xbsIndex_r4/AddSub  mode=Addition  use_carryin=off  use_carryout=off  en=off  latency=2  precision=User Defined  arith_type=Unsigned  n_bits=64  bin_pt=35  quantization=Truncate  overflow=Wrap  dbl_ovrd=off  use_behavioral_HDL=off  hw_selection=Fabric  pipelined=off  block_type=addsub
  AddSub1 : xbsIndex_r4/AddSub  mode=Addition  use_carryin=off  use_carryout=off  en=off  latency=2  precision=User Defined  arith_type=Unsigned  n_bits=64  bin_pt=35  quantization=Truncate  overflow=Wrap  dbl_ovrd=off  use_behavioral_HDL=off  hw_selection=Fabric  pipelined=off  block_type=addsub
  AddSub2 : xbsIndex_r4/AddSub  mode=Addition  use_carryin=off  use_carryout=off  en=off  latency=2  precision=User Defined  arith_type=Unsigned  n_bits=64  bin_pt=35  quantization=Truncate  overflow=Wrap  dbl_ovrd=off  use_behavioral_HDL=off  hw_selection=Fabric  pipelined=off  block_type=addsub
  pipeline243 : Subsystem  AncestorBlock=casper_library_delays/pipeline  mask(pipeline){latency=2}
      mask help:
      | An explicitly laid-out delay line to avoid mapping to SRL16s
      | for use in pipelining to help achieve timing closure.
      mask init:
      | pipeline_init(gcb,'latency',latency);
      settings: AttributesFormatString=Latency = %<latency>
      mask Display:
      | port_label('input', 1, 'd');
      | port_label('output', 1, 'q');
      | disp(['Z^-', num2str(latency)]);
  pipeline244 : Subsystem  AncestorBlock=casper_library_delays/pipeline  mask(pipeline){latency=2}
      mask help:
      | An explicitly laid-out delay line to avoid mapping to SRL16s
      | for use in pipelining to help achieve timing closure.
      mask init:
      | pipeline_init(gcb,'latency',latency);
      settings: AttributesFormatString=Latency = %<latency>
      mask Display:
      | port_label('input', 1, 'd');
      | port_label('output', 1, 'q');
      | disp(['Z^-', num2str(latency)]);
  pipeline{87,245,247,249} (4 alike) : casper_library_delays/pipeline  latency=3
      settings: AttributesFormatString=Latency = %<latency>
  pipeline246 : Subsystem  AncestorBlock=casper_library_delays/pipeline  mask(pipeline){latency=2}
      mask help:
      | An explicitly laid-out delay line to avoid mapping to SRL16s
      | for use in pipelining to help achieve timing closure.
      mask init:
      | pipeline_init(gcb,'latency',latency);
      settings: AttributesFormatString=Latency = %<latency>
      mask Display:
      | port_label('input', 1, 'd');
      | port_label('output', 1, 'q');
      | disp(['Z^-', num2str(latency)]);
  pipeline248 : Subsystem  AncestorBlock=casper_library_delays/pipeline  mask(pipeline){latency=2}
      mask help:
      | An explicitly laid-out delay line to avoid mapping to SRL16s
      | for use in pipelining to help achieve timing closure.
      mask init:
      | pipeline_init(gcb,'latency',latency);
      settings: AttributesFormatString=Latency = %<latency>
      mask Display:
      | port_label('input', 1, 'd');
      | port_label('output', 1, 'q');
      | disp(['Z^-', num2str(latency)]);
  Out1 : Outport
  wires:
  pipeline244/1(q) -> pipeline245/1
  pipeline243/1(q) -> pipeline87/1
  ch0/1 -> pipeline248/1(d)
  pipeline247/1 -> AddSub/2
  ch2/1 -> pipeline244/1(d)
  pipeline249/1 -> AddSub/1
  AddSub/1 -> AddSub2/1
  pipeline246/1(q) -> pipeline247/1
  pipeline248/1(q) -> pipeline249/1
  pipeline245/1 -> AddSub1/1
  AddSub2/1 -> Out1/1
  pipeline87/1 -> AddSub1/2
  AddSub1/1 -> AddSub2/2
  ch1/1 -> pipeline246/1(d)
  ch3/1 -> pipeline243/1(d)

== system doa_no_gotos/add_chanels5 ==
  ch0 : Inport
  ch1 : Inport  Port=2
  ch2 : Inport  Port=3
  ch3 : Inport  Port=4
  AddSub : xbsIndex_r4/AddSub  mode=Addition  use_carryin=off  use_carryout=off  en=off  latency=2  precision=User Defined  arith_type=Unsigned  n_bits=64  bin_pt=35  quantization=Truncate  overflow=Wrap  dbl_ovrd=off  use_behavioral_HDL=off  hw_selection=Fabric  pipelined=off  block_type=addsub
  AddSub1 : xbsIndex_r4/AddSub  mode=Addition  use_carryin=off  use_carryout=off  en=off  latency=2  precision=User Defined  arith_type=Unsigned  n_bits=64  bin_pt=35  quantization=Truncate  overflow=Wrap  dbl_ovrd=off  use_behavioral_HDL=off  hw_selection=Fabric  pipelined=off  block_type=addsub
  AddSub2 : xbsIndex_r4/AddSub  mode=Addition  use_carryin=off  use_carryout=off  en=off  latency=2  precision=User Defined  arith_type=Unsigned  n_bits=64  bin_pt=35  quantization=Truncate  overflow=Wrap  dbl_ovrd=off  use_behavioral_HDL=off  hw_selection=Fabric  pipelined=off  block_type=addsub
  pipeline243 : Subsystem  AncestorBlock=casper_library_delays/pipeline  mask(pipeline){latency=2}
      mask help:
      | An explicitly laid-out delay line to avoid mapping to SRL16s
      | for use in pipelining to help achieve timing closure.
      mask init:
      | pipeline_init(gcb,'latency',latency);
      settings: AttributesFormatString=Latency = %<latency>
      mask Display:
      | port_label('input', 1, 'd');
      | port_label('output', 1, 'q');
      | disp(['Z^-', num2str(latency)]);
  pipeline244 : Subsystem  AncestorBlock=casper_library_delays/pipeline  mask(pipeline){latency=2}
      mask help:
      | An explicitly laid-out delay line to avoid mapping to SRL16s
      | for use in pipelining to help achieve timing closure.
      mask init:
      | pipeline_init(gcb,'latency',latency);
      settings: AttributesFormatString=Latency = %<latency>
      mask Display:
      | port_label('input', 1, 'd');
      | port_label('output', 1, 'q');
      | disp(['Z^-', num2str(latency)]);
  pipeline{87,245,247,249} (4 alike) : casper_library_delays/pipeline  latency=3
      settings: AttributesFormatString=Latency = %<latency>
  pipeline246 : Subsystem  AncestorBlock=casper_library_delays/pipeline  mask(pipeline){latency=2}
      mask help:
      | An explicitly laid-out delay line to avoid mapping to SRL16s
      | for use in pipelining to help achieve timing closure.
      mask init:
      | pipeline_init(gcb,'latency',latency);
      settings: AttributesFormatString=Latency = %<latency>
      mask Display:
      | port_label('input', 1, 'd');
      | port_label('output', 1, 'q');
      | disp(['Z^-', num2str(latency)]);
  pipeline248 : Subsystem  AncestorBlock=casper_library_delays/pipeline  mask(pipeline){latency=2}
      mask help:
      | An explicitly laid-out delay line to avoid mapping to SRL16s
      | for use in pipelining to help achieve timing closure.
      mask init:
      | pipeline_init(gcb,'latency',latency);
      settings: AttributesFormatString=Latency = %<latency>
      mask Display:
      | port_label('input', 1, 'd');
      | port_label('output', 1, 'q');
      | disp(['Z^-', num2str(latency)]);
  Out1 : Outport
  wires:
  pipeline244/1(q) -> pipeline245/1
  pipeline243/1(q) -> pipeline87/1
  ch0/1 -> pipeline248/1(d)
  pipeline247/1 -> AddSub/2
  ch2/1 -> pipeline244/1(d)
  pipeline249/1 -> AddSub/1
  AddSub/1 -> AddSub2/1
  pipeline246/1(q) -> pipeline247/1
  pipeline248/1(q) -> pipeline249/1
  pipeline245/1 -> AddSub1/1
  AddSub2/1 -> Out1/1
  pipeline87/1 -> AddSub1/2
  AddSub1/1 -> AddSub2/2
  ch1/1 -> pipeline246/1(d)
  ch3/1 -> pipeline243/1(d)
